simulink model "MODELO_PELICAN_2025"  (R2025a)
settings: Solver=VariableStepAuto  StartTime=0.0  StopTime=0.3  RelTol=1e-3
settings Model: Creator=juanduque  LastModifiedBy=rsp
settings SolverCC: AlgebraicLoopSolver=TrustRegion
settings DataIOCC: ReturnWorkspaceOutputs=off
settings OptimizationCC: ReuseModelBlockBuffer=off
settings DebuggingCC: UnconnectedInputMsg=warning  UnconnectedOutputMsg=warning  UnconnectedLineMsg=warning  ArithmeticOperatorsInVariantConditions=warning
settings ModelReferenceCC: EnableRefExpFcnMdlSchedulingChecks=on
settings SFSimCC: SimUseLocalCustomCode=off  CustomCodeUndefinedFunction=UseInterfaceOnly
settings RTWCC: RTWUseLocalCustomCode=off  GPUComputeCapability=3.5
settings CodeAppCC: StateflowObjectComments=on

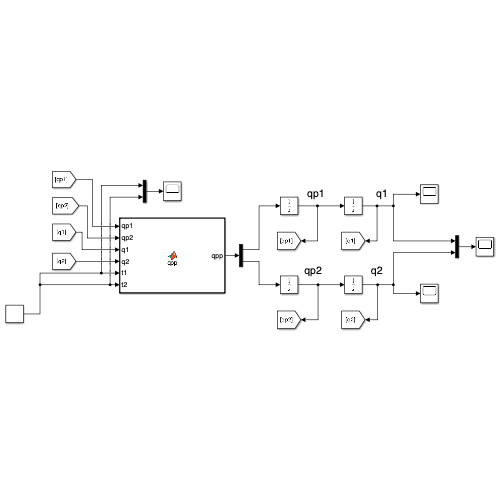
[thumbnail: Simulink's stored preview of the top-level diagram]
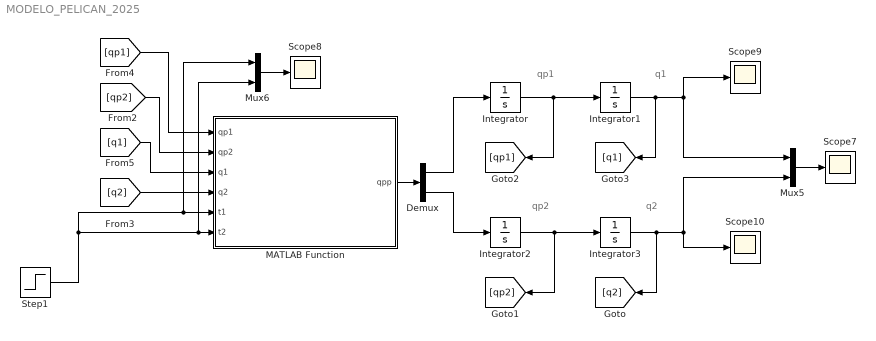
== system MODELO_PELICAN_2025 ==
  note: q2
  note: q1
  note: qp2
  note: qp1
  Demux : Demux  Outputs=2
  Integrator : Integrator
  Integrator1 : Integrator  InitialCondition=pi/10
  Integrator2 : Integrator
  Integrator3 : Integrator  InitialCondition=pi/30
  MATLAB Function : MATLAB Function  TreatAsAtomicUnit=on
  Mux5 : Mux  Inputs=2
  Mux6 : Mux  Inputs=2
  Scope{7..10} (4 alike) : Scope
      Scope10 settings: ActiveDisplayYMinimum=0.08832  ActiveDisplayYMaximum=0.25232  DataLoggingVariableName=ScopeData7
      Scope7 settings: ActiveDisplayYMinimum=-1.66183  ActiveDisplayYMaximum=3.79215  DataLoggingVariableName=ScopeData4
      Scope8 settings: ActiveDisplayYMinimum=-612.89283  ActiveDisplayYMaximum=201.36568  DataLoggingVariableName=ScopeData5
      Scope9 settings: ActiveDisplayYMinimum=-0.36732  ActiveDisplayYMaximum=0.38988  DataLoggingVariableName=ScopeData6
  Step1 : Step  Time=0  After=0  SampleTime=0
  wires:
  Integrator1/1 -> [q1], Scope9/1, Mux5/1
  Demux/2 -> Integrator2/1
  Integrator2/1 -> Integrator3/1, [qp2]
  [qp2] -> MATLAB Function/2(qp2)
  MATLAB Function/1(qpp) -> Demux/1
  Integrator3/1 -> [q2], Scope10/1, Mux5/2
  [qp1] -> MATLAB Function/1(qp1)
  [q2] -> MATLAB Function/4(q2)
  Mux6/1 -> Scope8/1
  Demux/1 -> Integrator/1
  Mux5/1 -> Scope7/1
  Step1/1 -> Mux6/1, MATLAB Function/5(t1), Mux6/2, MATLAB Function/6(t2)
  Integrator/1 -> Integrator1/1, [qp1]
  [q1] -> MATLAB Function/3(q1)

== matlab function MODELO_PELICAN_2025/MATLAB Function ==
  data: qp1 input; qp2 input; q1 input; q2 input; t1 input; t2 input; qpp output
function qpp = qpp(qp1, qp2, q1, q2, t1, t2)

% Parametros del robot
m1=23.902; m2=3.88;
L1=0.45; L2=0.45; lc1=0.091;lc2=0.0229;
I1=1.266; I2=0.093;

%Matriz de masas
m11= m1*lc1^2 + m2*(L1^2 +lc2^2+2*L1*lc2*cos(q2))+I1+I2;
m12=m2*(lc2^2 +L1*lc2*cos(q2))+I2;
m21=m2*(lc2^2+L1*lc2*cos(q2))+I2
m22=m2*lc2^2+I2;
M=[ m11 m12; m21 m22];
%Matriz de Coriolis
c11=-m2*L1*lc2*sin(q2)*qp2;
c12=-m2*L1*lc2*sin(q2)*(qp1+qp2);
c21=m2*L1*lc2*sin(q2)*qp1;
c22=0;
C=[c11 c12; c21 c22];
%Vector de gravedad
g1=(m1*lc1+m2*L1)*9.8*sin(q1)+m2*lc2*9.8*sin(q1+q2);
g2=m2*lc2*9.8*sin(q1+q2);
G=[g1 g2]';
T=[t1 t2]';
q=[q1  q2]';
qp=[qp1 qp2]';
%calculo de la aceleracion
qpp=[inv(M)*(T-C*qp-G)];
qpp1=qpp(1,1);
qpp2=qpp(2,1);

qpp = [qpp1; qpp2];
